simulink model "picpicpic_org"  (Simulink 10.0)
settings: Solver=FixedStepAuto  StartTime=0.0  StopTime=20  RelTol=1e-3
libraries: instrumentlib x3, visionsources x1
settings Model: Creator=sbuadu  LastModifiedBy=annonymous
settings DataIOCC: SaveFormat=Dataset
settings OptimizationCC: LifeSpan=auto
settings DebuggingCC: UnderspecifiedInitializationDetection=Simplified  MergeDetectMultiDrivingBlocksExec=error  SFUnexpectedBacktrackingDiag=error  SFNoUnconditionalDefaultTransitionDiag=error  SFExecutionAtInitializationDiag=warning
settings HardwareCC: ProdBitPerPointer=64  ProdBitPerSizeT=64  ProdBitPerPtrDiffT=64  ProdLargestAtomicFloat=Float  ProdIntDivRoundTo=Zero  ProdEndianess=LittleEndian  ProdWordSize=64  ProdHWDeviceType=Intel->x86-64 (Windows64)
settings ModelReferenceCC: PropagateSignalLabelsOutOfModel=on
settings GRTTargetCC: TargetLangStandard=C99 (ISO)  CombineOutputUpdateFcns=on  GRTInterface=off
settings ConfigComp: CovMetricSettings=dwe  CovHtmlReporting=off  CovSaveCumulativeToWorkspaceVar=off  CovSaveSingleToWorkspaceVar=off

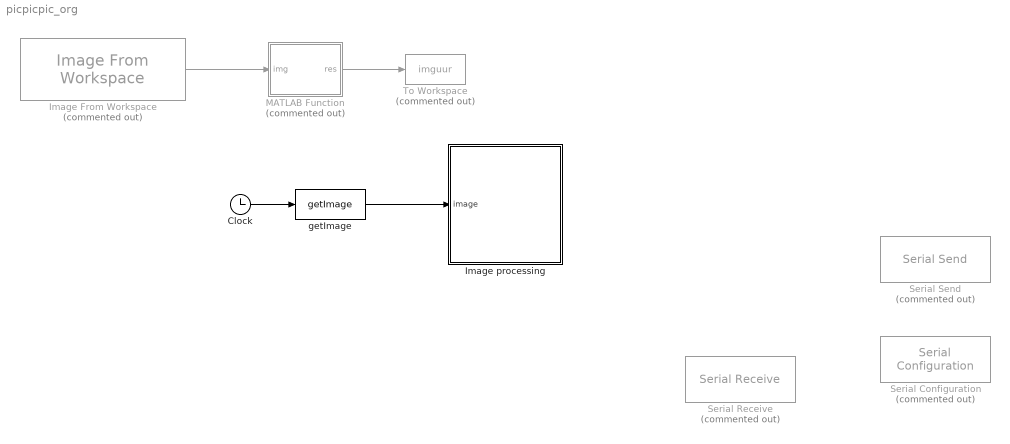
== system picpicpic_org ==
  Clock : Clock
  Image From Workspace : visionsources/Image From Workspace  Tag=vipblks_nd  Commented=on  ImageValue=image  Ts=5  imagePorts=One multidimensional signal  OutPortLabels=R|G|B  ImageDataType=Inherit from 'Value'  Signed=on  WordLength=16  sdImageDataType=sfix(16)  FractionLengthMode=User-defined  FractionLength=15
      settings: SourceProductName=Computer Vision Toolbox  SourceProductBaseCode=VP
  Image processing : Subsystem
  MATLAB Function : MATLAB Function  Commented=on  TreatAsAtomicUnit=on
  Serial Configuration : instrumentlib/Serial Configuration  Priority=-200000  Commented=on  ComPortMenu=<Please select a port...>  ComPort=<Please select a port...>  BaudRate=9600  DataBits=8  Parity=none  StopBits=1  FlowControl=none  Timeout=10  ByteOrder=LittleEndian
  Serial Receive : instrumentlib/Serial Receive  Commented=on  ComPortMenu=<Please select a port...>  ComPort=<Please select a port...>  Terminator=<none>  DataSize=[1 1]  DataType=uint8  EnableBlockingMode=on  ActionDataUnavailable=Output last received value  CustomValue=0  SampleTime=0.01
  Serial Send : instrumentlib/Serial Send  Commented=on  ComPortMenu=<Please select a port...>  ComPort=<Please select a port...>  Terminator=<none>  EnableBlockingMode=on
  To Workspace : ToWorkspace  Commented=on  VariableName=imguur  SaveFormat=Structure With Time  SampleTime=-1
      settings: Save2DSignal=2-D array (concatenate along first dimension)
  getImage : MATLABFcn  MATLABFcn=getImage  Output1D=off
  wires:
  Image From Workspace/1 -> MATLAB Function/1(img)
  MATLAB Function/1(res) -> To Workspace/1
  getImage/1 -> Image processing/1("image ")
  Clock/1 -> getImage/1

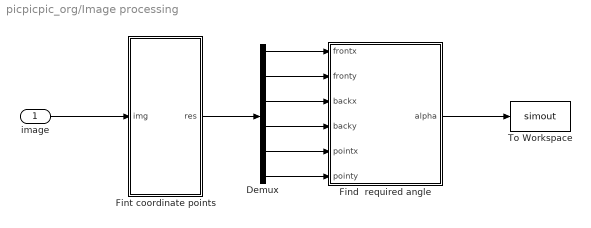
== system picpicpic_org/Image processing ==
  "image " : Inport
  Demux : Demux  Outputs=6
  Find  required angle : MATLAB Function  TreatAsAtomicUnit=on
  Fint coordinate points : MATLAB Function  TreatAsAtomicUnit=on
  To Workspace : ToWorkspace  VariableName=simout  SaveFormat=Timeseries  SampleTime=-1
  wires:
  Demux/2 -> Find  required angle/2(fronty)
  Demux/4 -> Find  required angle/4(backy)
  Demux/1 -> Find  required angle/1(frontx)
  Demux/3 -> Find  required angle/3(backx)
  Demux/5 -> Find  required angle/5(pointx)
  Demux/6 -> Find  required angle/6(pointy)
  "image "/1 -> Fint coordinate points/1(img)
  Fint coordinate points/1(res) -> Demux/1
  Find  required angle/1(alpha) -> To Workspace/1

== matlab function Image processing/Fint coordinate points ==
  data: img input double; res output double
function res = findColor(img)
% image is a 480 x 1920 matrix. image = [r g b] where r,g,b (480X640) 
resizeIm = 0.1;

%image = ('double1.jpg');
%image = imread(image);
C = uint8(zeros(480,640,3));
C(:,:,1) = img(:,1:640);
C(:,:,2) = img(:,641:1280);
C(:,:,3) = img(:,1281:1920);

image = imresize(C,resizeIm);
[m,n] = size(image);
disp('m:');
disp(m);
disp('n:');
disp(n);

% red = image(:,1:640);
% %green = image(:,641:1280);
% blue = image(:,1281:1920);
% green = image - red; 

red = image(:,:,1);
blue = image(:,:,3);
red_temp = uint8(zeros(48,64,3));
red_temp(:,:,1)= red;
red_temp(:,:,2)= red;
red_temp(:,:,3)= red;
green = image - red_temp; 

greenIntensity = rgb2gray(green);
greenBinary = imbinarize(greenIntensity);
s = regionprops(greenBinary,'centroid');
centroids = cat(1, s.Centroid);
a = regionprops(greenBinary, 'area');
area = cat(1, a.Area);

imshow(greenBinary); 
if (centroids ~= 0 )
    hold on
    plot(centroids(:,1),centroids(:,2), 'b*')
    hold off
end 


[sortedValues,sortIndex] = sort(area(:),'descend');

if size(area,1) == 2
    frontPos = centroids(sortIndex(1),:);
    backPos = centroids(sortIndex(2),:);
    destination = [0,0];
elseif size(area,1)== 3
    destination = centroids(sortIndex(1),:);
    frontPos = centroids(sortIndex(2),:);
    backPos = centroids(sortIndex(3),:);
else
    error('did not find correct number of green spots');
end
    res = [frontpos, frontpos1, backpos,backpos1, destination,destination1]  ; 

end

== matlab function Image processing/Find required angle ==
  data: frontx input double; fronty input double; backx input double; backy input double; pointx input double; pointy input double; alpha output double
function alpha = findAngle(frontx, fronty, backx, backy, pointx, pointy)

%%setting the coordinates for the middle of the car 
if frontx < backx
    carx = frontx + abs(backx - frontx)/2; 
else
    carx = backx + abs(backx - frontx)/2; 
end

if fronty < backy
    cary = fronty + abs(backy - fronty)/2; 
else
    cary = backy + abs(backy - fronty)/2;  
end


%%finding the vector between car and destination 
deltax = pointx - carx; 
deltay = pointy-cary; 
delta = [deltax deltay]; 
%%tvector from rotation point to frot of vehicle
betax = frontx - carx;
betay = fronty-cary; 
beta = [betax betay]; 

alpha = atan2(beta(2), beta(1)) - atan2(delta(2), delta(1)); 

alpha = alpha*180/pi; 

if alpha > 180
alpha = alpha - 360; 
end


end

== matlab function MATLAB Function ==
  data: res output double; img input double
function res = fcn(img)

res = 0; 

r = img(:,:,1); 
g = img(:,:,2); 
b = img(:,:,3)

image(:,:,1) = r;
image(:,:,2) = g;
image(:,:,3) = b;
resizeIm = 0.1;

[m,n] = size(image);

red = image(:,:,1);
blue = image(:,:,3);
green = image - red;
greenIntensity = rgb2gray(green);
greenBinary = imbinarize(greenIntensity);
s = regionprops(greenBinary,'centroid');
centroids = cat(1, s.Centroid);
a = regionprops(greenBinary, 'area');
area = cat(1, a.Area);

disp('Hello')
figure;
imshow(greenBinary);
hold on
plot(centroids(:,1),centroids(:,2), 'b*')
hold off
disp('Hello')

[sortedValues,sortIndex] = sort(area(:),'descend');

if size(area,1) == 2
    frontPos = centroids(sortIndex(1),:);
    backPos = centroids(sortIndex(2),:);
    destination = [0,0];
    disp('Hello')
elseif size(area,1)== 3
    destination = centroids(sortIndex(1),:);
    frontPos = centroids(sortIndex(2),:);
    backPos = centroids(sortIndex(3),:);
    disp('Hello')
else
    frontPos = [0, 0];
    backPos = [0,0];
    destination = [0,0];
    disp('didnt findHello')
    
end
res = [frontPos(1), frontPos(2), backPos(1),backPos(2), destination(1),destination(2)]

end
